simulink model "COAP_Client_GetPut"  (R2017b)
settings: Solver=FixedStepDiscrete  StartTime=0.0  StopTime=10.0  FixedStep=1e-3  RelTol=1e-3
libraries: mbed_ethernet_coap x5, mbed_lib x3, BTN_lib x1, mbed_ethernet x1
settings Model: Creator=Anwender  LastModifiedBy=oh
settings DataIOCC: LimitDataPoints=on  SaveFormat=Array
settings OptimizationCC: LifeSpan=1
settings DebuggingCC: SFUnexpectedBacktrackingDiag=warning  SFNoUnconditionalDefaultTransitionDiag=warning  SFExecutionAtInitializationDiag=none
settings HardwareCC: ProdBitPerPointer=32  ProdBitPerSizeT=32  ProdBitPerPtrDiffT=32  ProdLargestAtomicInteger=Long  ProdLargestAtomicFloat=Double  ProdIntDivRoundTo=Undefined  ProdWordSize=32  ProdHWDeviceType=ARM Compatible->ARM Cortex
settings ModelReferenceCC: PropagateSignalLabelsOutOfModel=off
settings SFSimCC: MATLABDynamicMemAlloc=off
settings RTWCC: SystemTargetFile=mbed.tlc  TemplateMakefile=mbed.tmf  Description=Mbed Target (Embedded Target)  TargetLang=C++
settings CodeAppCC: IgnoreCustomStorageClasses=off  StateflowObjectComments=on
settings STFCustomTargetCC: TargetLibSuffix=.a  GenerateSampleERTMain=on  CombineOutputUpdateFcns=on  ERTCustomFileBanners=on  SupportContinuousTime=off  SupportNonInlinedSFcns=off  RemoveResetFunc=on  MATLABClassNameForMDSCustomization=Simulink.SoftwareTarget.ERTCustomization  ModelStepFunctionPrototypeControlCompliant=on  GRTInterface=off  SystemTargetFile=mbed.tlc
settings ERTTargetCC: MultiwordLength=2048  GenerateSampleERTMain=on  ParMdlRefBuildCompliant=off  CompOptLevelCompliant=off  ConcurrentExecutionCompliant=off  CPPClassGenCompliant=off  UseToolchainInfoCompliant=off  ERTCustomFileTemplate=mbed_file_process.tlc  ConvertIfToSwitch=off  SuppressUnreachableDefaultCases=off
settings ConfigComp: CovMetricSettings=dw  CovHtmlReporting=on  CovSaveCumulativeToWorkspaceVar=on  CovSaveSingleToWorkspaceVar=on  CovExternalEMLEnable=off

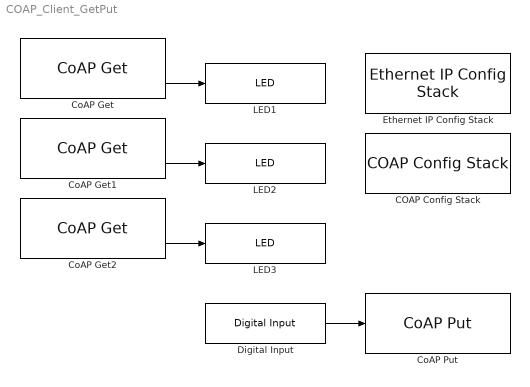
== system COAP_Client_GetPut ==
  COAP Config Stack : mbed_ethernet_coap/COAP Config Stack  Priority=0  ip_addr=10.10.199.171
      settings: SourceProductName=Mbed Target
  CoAP Get : mbed_ethernet_coap/CoAP Get  Priority=0  token=1  path=/LED1  method=COAP_MSG_CODE_REQUEST_GET  SampleTime=[1,0.2]
      settings: SourceProductName=Mbed Target
  CoAP Get1 : mbed_ethernet_coap/CoAP Get  Priority=0  token=2  path=/LED2  method=COAP_MSG_CODE_REQUEST_GET  SampleTime=[1,0.4]
      settings: SourceProductName=Mbed Target
  CoAP Get2 : mbed_ethernet_coap/CoAP Get  Priority=0  token=3  path=/LED3  method=COAP_MSG_CODE_REQUEST_GET  SampleTime=[1,0.6]
      settings: SourceProductName=Mbed Target
  CoAP Put : mbed_ethernet_coap/CoAP Put  Priority=0  token=4  path=/Button  method=COAP_MSG_CODE_REQUEST_PUT  SampleTime=[1,0.8]
      settings: SourceProductName=Mbed Target
  Digital Input : BTN_lib/Digital Input  SampleTime=0.25
  Ethernet IP Config Stack : mbed_ethernet/Ethernet IP Config Stack  Priority=1  sDHCP=off  DHCP=0  ip_addr=192.168.0.1  sub_mask=255.255.255.0  gateway=0.0.0.0  SerialDebugInfo=off
      settings: SourceProductName=Mbed Target
  LED1 : mbed_lib/GPIO/LED  nLED=1  SampleTime=0.5
      settings: SourceProductName=Mbed Target
  LED2 : mbed_lib/GPIO/LED  nLED=2  SampleTime=0.5
      settings: SourceProductName=Mbed Target
  LED3 : mbed_lib/GPIO/LED  nLED=3  SampleTime=0.5
      settings: SourceProductName=Mbed Target
  wires:
  CoAP Get/2 -> LED1/1
  CoAP Get1/2 -> LED2/1
  CoAP Get2/2 -> LED3/1
  Digital Input/1 -> CoAP Put/1
